simulink model "balancing_robot"  (R2020b)
settings: Solver=VariableStepAuto  StartTime=0.0  StopTime=10.0  RelTol=1e-3
settings Model: Creator=utente  LastModifiedBy=utente

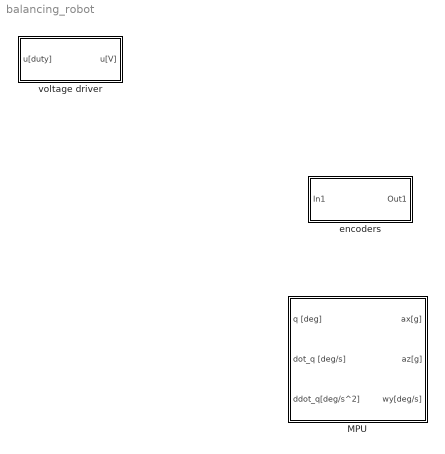
== system balancing_robot ==
  MPU : Subsystem
  encoders : Subsystem
  voltage driver : Subsystem

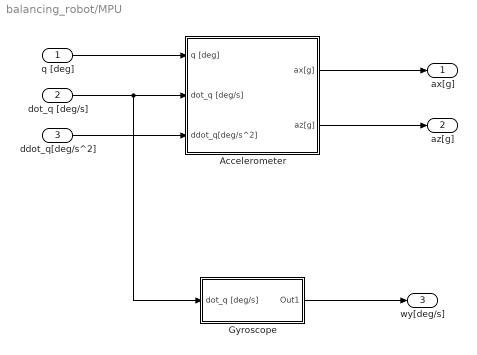
== system balancing_robot/MPU ==
  q [deg] : Inport
  dot_q [deg/s] : Inport  Port=2
  ddot_q[deg/s^2] : Inport  Port=3
  Accelerometer : Subsystem
  Gyroscope : Subsystem
  ax[g] : Outport
  az[g] : Outport  Port=2
  wy[deg/s] : Outport  Port=3
  wires:
  q [deg]/1 -> Accelerometer/1(q [deg])
  dot_q [deg/s]/1 -> Gyroscope/1(dot_q [deg/s]), Accelerometer/2(dot_q [deg/s])
  ddot_q[deg/s^2]/1 -> Accelerometer/3(ddot_q[deg/s^2])
  Gyroscope/1(Out1) -> wy[deg/s]/1
  Accelerometer/1(ax[g]) -> ax[g]/1
  Accelerometer/2(az[g]) -> az[g]/1

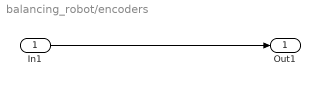
== system balancing_robot/encoders ==
  In1 : Inport
  Out1 : Outport
  wires:
  In1/1 -> Out1/1

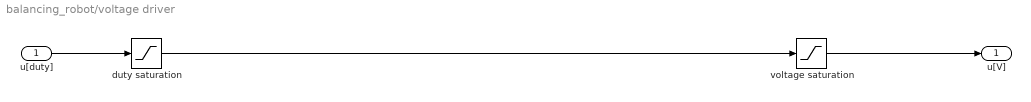
== system balancing_robot/voltage driver ==
  u[duty] : Inport
  duty saturation : Saturate
  voltage saturation : Saturate
  u[V] : Outport
  wires:
  u[duty]/1 -> duty saturation/1
  voltage saturation/1 -> u[V]/1
  duty saturation/1 -> voltage saturation/1

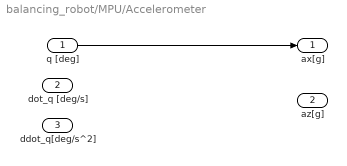
== system balancing_robot/MPU/Accelerometer ==
  q [deg] : Inport
  dot_q [deg/s] : Inport  Port=2
  ddot_q[deg/s^2] : Inport  Port=3
  ax[g] : Outport
  az[g] : Outport  Port=2
  wires:
  q [deg]/1 -> ax[g]/1

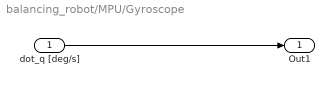
== system balancing_robot/MPU/Gyroscope ==
  dot_q [deg/s] : Inport
  Out1 : Outport
  wires:
  dot_q [deg/s]/1 -> Out1/1
